simulink model "Copy_of_canceshi"  (Simulink 7.6)
settings: Solver=ode4  StartTime=0.0  StopTime=inf  FixedStep=0.1  RelTol=1e-3
undefined symbols (not defined in the file or in its folder): bit, Standard
libraries: xpclib x5
CloseFcn:
  | rtwprivate ssgencode ModelCloseRequest canceshi
settings Model: xpc_rtwmakecfg_data=_xpccanac2pci_  Creator=Administrator  LastModifiedBy=Administrator  SimulationMode=external  BufferReuse=off
settings OptimizationCC: BlockReduction=off  OptimizeBlockIOStorage=off  BufferReuse=off  ExpressionFolding=off  LocalBlockOutputs=off
settings HardwareCC: ProdIntDivRoundTo=Zero  ProdEndianess=LittleEndian  ProdHWDeviceType=Generic->32-bit x86 compatible
settings RTWCC: SystemTargetFile=xpctarget.tlc  TemplateMakefile=xpc_default_tmf  Description=xPC Target  ProcessScript=xpctarget_make_rtw_hook  RTWCompilerOptimization=On
settings xpcTargetCC: TargetFcnLib=ansi_tfl_table_tmw.mat  TargetFunctionLibrary=XPC_BLAS  ERTCodeCoverageTool=None  ParMdlRefBuildCompliant=on  CombineSignalStateStructs=off  PortableWordSizes=off  xPCLoadParamSetFile=off  xPCConcurrentTasks=off  xPCEnableSFAnimation=off

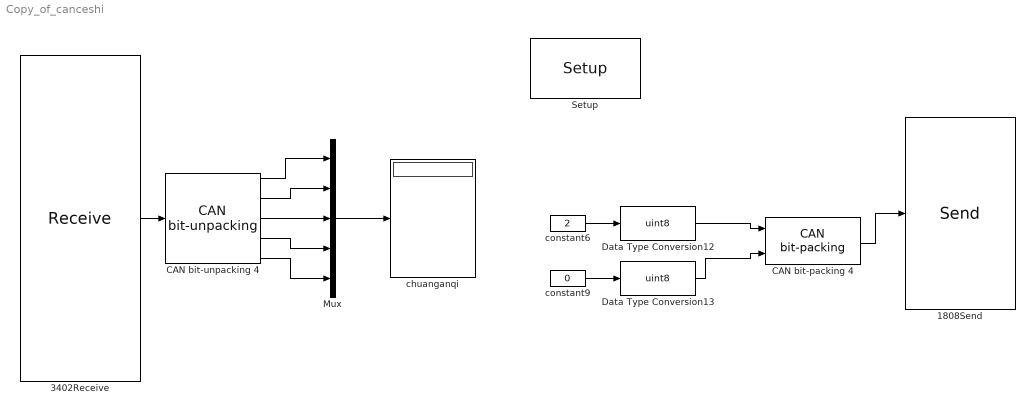
== system Copy_of_canceshi ==
  1808Send : xpclib/CAN/Softing/CAN-AC2-PCI SJA 1000/Send   board=1  canPort=CAN 2  range=Standard (11-bit)  ids=3  sizes=[8]  output=off  ts=-1  ididx=[0]
  "3402Receive " : xpclib/CAN/Softing/CAN-AC2-PCI SJA 1000/Receive   board=1  canPort=CAN 2  range=Standard (11-bit)  ids=3  lengths=8  output=Data  inten=off  ts=-1  ididx=[0]
  CAN bit-packing 4 : xpclib/CAN/Utilities/CAN bit-packing   bitpatterns={ [0:7] [8:15] }
  CAN bit-unpacking 4 : xpclib/CAN/Utilities/CAN bit-unpacking   bitpatterns={ [0:7],[8:15],[16:23],[24:31],[32:39]}  dtypes={ 'uint8','uint8','uint8','uint8','uint8' }
  Data Type Conversion12 : DataTypeConversion  OutDataTypeStr=uint8
  Data Type Conversion13 : DataTypeConversion  OutDataTypeStr=uint8
  Mux : Mux  Inputs=5
  "Setup " : xpclib/CAN/Softing/CAN-AC2-PCI SJA 1000/Setup   board=1  can1bus=Highspeed (ISO 11898)  can1Baudrate=500 kBaud  can1UserBR=[1,1,4,3]  can2bus=Highspeed (ISO 11898)  can2Baudrate=500 kBaud  can2UserBR=[1,1,4,3]  init=[]  term=[]  bus_off_out=off  bus_off_rec=Off  ioBaseAddress=-1
  chuanganqi : Display
  constant6 : Constant  Value=2
  constant9 : Constant  Value=0
  wires:
  "3402Receive "/1 -> CAN bit-unpacking 4/1
  CAN bit-unpacking 4/1 -> Mux/1
  Mux/1 -> chuanganqi/1
  constant6/1 -> Data Type Conversion12/1
  Data Type Conversion12/1 -> CAN bit-packing 4/1
  Data Type Conversion13/1 -> CAN bit-packing 4/2
  constant9/1 -> Data Type Conversion13/1
  CAN bit-packing 4/1 -> 1808Send/1
  CAN bit-unpacking 4/5 -> Mux/5
  CAN bit-unpacking 4/4 -> Mux/4
  CAN bit-unpacking 4/3 -> Mux/3
  CAN bit-unpacking 4/2 -> Mux/2
